simulink model "Exercitiul4_2"  (R2016a)
settings: Solver=VariableStepDiscrete  StartTime=0.0  StopTime=168  RelTol=1e-3
undefined symbols (not defined in the file): m, n
settings Model: Creator=Cristina  LastModifiedBy=Cristina

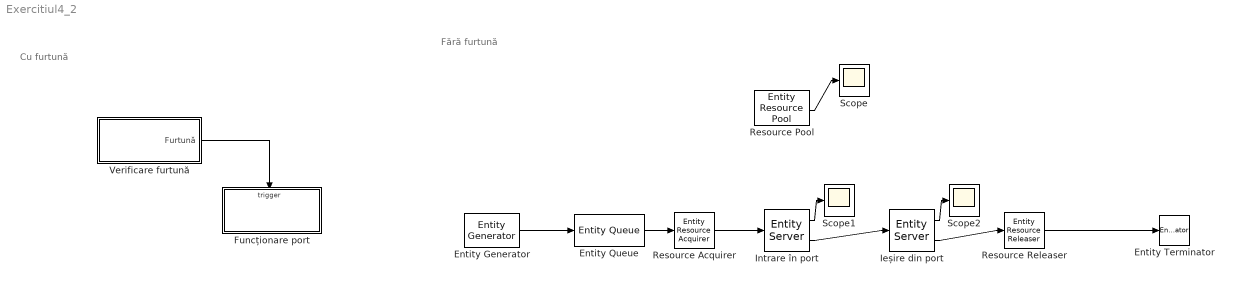
== system Exercitiul4_2 ==
  note: Fără furtună
  note: Cu furtună
  Entity Generator : EntityGenerator  OutputPortMessageModes=m  TimeSource=MATLAB action  IntergenerationTimeAction=dt = rand(1.7 + 3 * rand);  EntityType=Structured  EntityTypeName=Entity
  Entity Queue : EntityQueue  InputPortMessageModes=m  OutputPortMessageModes=m
      settings: OutputPortMap=o5
  Entity Terminator : EntityTerminator  InputPortMessageModes=m
  Funcționare port : Subsystem  TreatAsAtomicUnit=on
  Ieșire din port : EntityServer  InputPortMessageModes=m  OutputPortMessageModes=n,m  Capacity=3  ServiceTimeValue=0.25  ServiceTimeAction=dt = 7.4 + 3 * rand;  AverageWait=on
      settings: OutputPortMap=o4,o9
  Intrare în port : EntityServer  InputPortMessageModes=m  OutputPortMessageModes=n,m  Capacity=3  ServiceTimeSource=MATLAB action  ServiceTimeAction=dt = 6.9 + 3 * rand;  AverageWait=on
      settings: OutputPortMap=o4,o9
  Resource Acquirer : EntityResourceAcquirer  InputPortMessageModes=m  OutputPortMessageModes=m  NumberWaitingEntities=5  ResourceName=Dane
      settings: OutputPortMap=o3
  Resource Releaser : EntityResourceReleaser  InputPortMessageModes=m  OutputPortMessageModes=m  ResourceToRelease=Selected  ResourceName=Dane
  Resource Pool : EntityResourcePool  ResourceName=Dane  ResourceAmount=3  AverageUtilization=on
      settings: OutputPortMap=o1
  Scope : Scope
  Scope1 : Scope
  Scope2 : Scope
  Verificare furtună : Subsystem
  wires:
  Verificare furtună/1(Furtună) -> Funcționare port/Trigger
  Entity Queue/1 -> Resource Acquirer/1
  Entity Generator/1 -> Entity Queue/1
  Ieșire din port/2 -> Resource Releaser/1
  Intrare în port/2 -> Ieșire din port/1
  Resource Acquirer/1 -> Intrare în port/1
  Resource Releaser/1 -> Entity Terminator/1
  Intrare în port/1 -> Scope1/1
  Ieșire din port/1 -> Scope2/1
  Resource Pool/1 -> Scope/1

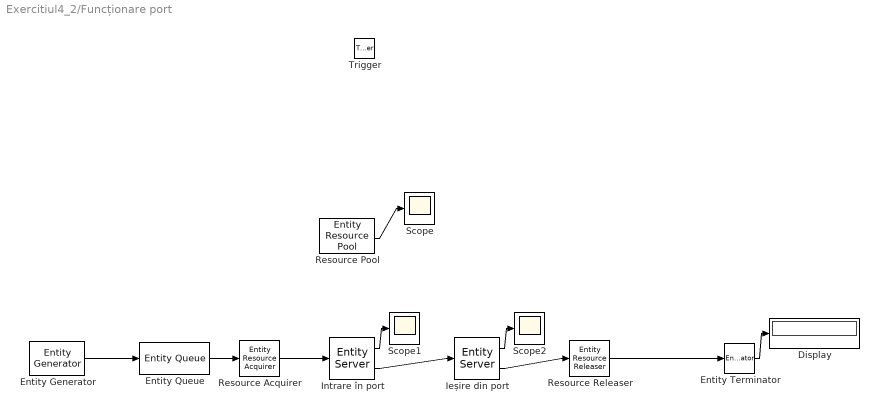
== system Exercitiul4_2/Funcționare port ==
  Trigger : TriggerPort  VariantControl=Variant
  Display : Display
  Entity Generator : EntityGenerator  OutputPortMessageModes=m  TimeSource=MATLAB action  IntergenerationTimeAction=dt = rand(1.7 + 3 * rand);  EntityType=Structured  EntityTypeName=Entity
  Entity Queue : EntityQueue  InputPortMessageModes=m  OutputPortMessageModes=m
      settings: OutputPortMap=o5
  Entity Terminator : EntityTerminator  InputPortMessageModes=m  NumberEntitiesArrived=on
      settings: OutputPortMap=o0
  Ieșire din port : EntityServer  InputPortMessageModes=m  OutputPortMessageModes=n,m  Capacity=3  ServiceTimeValue=0.25  ServiceTimeAction=dt = 7.4 + 3 * rand;  AverageWait=on
      settings: OutputPortMap=o4,o9
  Intrare în port : EntityServer  InputPortMessageModes=m  OutputPortMessageModes=n,m  Capacity=3  ServiceTimeSource=MATLAB action  ServiceTimeAction=dt = 7.4 + 3 * rand;  AverageWait=on
      settings: OutputPortMap=o4,o9
  Resource Acquirer : EntityResourceAcquirer  InputPortMessageModes=m  OutputPortMessageModes=m  NumberWaitingEntities=5  ResourceName=Dane
      settings: OutputPortMap=o3
  Resource Releaser : EntityResourceReleaser  InputPortMessageModes=m  OutputPortMessageModes=m  ResourceToRelease=Selected  ResourceName=Dane
  Resource Pool : EntityResourcePool  ResourceName=Dane  ResourceAmount=3  AverageUtilization=on
      settings: OutputPortMap=o1
  Scope : Scope
  Scope1 : Scope
  Scope2 : Scope
  wires:
  Entity Queue/1 -> Resource Acquirer/1
  Entity Generator/1 -> Entity Queue/1
  Ieșire din port/2 -> Resource Releaser/1
  Intrare în port/2 -> Ieșire din port/1
  Resource Acquirer/1 -> Intrare în port/1
  Resource Releaser/1 -> Entity Terminator/1
  Intrare în port/1 -> Scope1/1
  Ieșire din port/1 -> Scope2/1
  Resource Pool/1 -> Scope/1
  Entity Terminator/1 -> Display/1

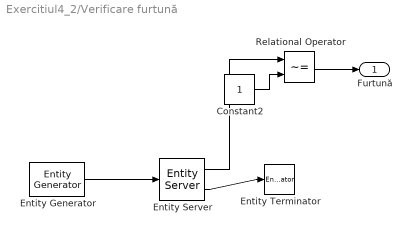
== system Exercitiul4_2/Verificare furtună ==
  Constant2 : Constant
  Entity Generator : EntityGenerator  OutputPortMessageModes=m  TimeSource=MATLAB action  IntergenerationTimeAction=dt = 44 + 8*rand;  EntityType=Structured  EntityTypeName=Entity
  Entity Server : EntityServer  InputPortMessageModes=m  OutputPortMessageModes=n,m  Capacity=1  ServiceTimeSource=MATLAB action  ServiceTimeAction=dt = 2 + 4*rand;  NumberEntitiesInBlock=on
      settings: OutputPortMap=o1,o9
  Entity Terminator : EntityTerminator  InputPortMessageModes=m
  Relational Operator : RelationalOperator  Operator=~=  OutDataTypeStr=boolean
  Furtună : Outport
  wires:
  Entity Generator/1 -> Entity Server/1
  Entity Server/2 -> Entity Terminator/1
  Constant2/1 -> Relational Operator/2
  Relational Operator/1 -> Furtună/1
  Entity Server/1 -> Relational Operator/1
